simulink model "complementary_controller"  (R2013a)
settings: Solver=ode3  StartTime=0.0  StopTime=15  FixedStep=0.004  RelTol=1e-3
undefined symbols (not defined in the file or in its folder): DiscIntNeverNeededParam, sigbuilder_block
libraries: simulink x3
settings Model: Creator=Matthias  LastModifiedBy=Matthias
settings OptimizationCC: InlineParams=on  InlineInvariantSignals=on  EnhancedBackFolding=on  EfficientFloat2IntCast=on
settings HardwareCC: ProdLargestAtomicInteger=Long  ProdLargestAtomicFloat=Double  ProdHWDeviceType=ARM Compatible->ARM Cortex
settings ModelReferenceCC: UpdateModelReferenceTargets=IfOutOfDate
settings SFSimCC: SFSimEcho=off
settings RTWCC: GenCodeOnly=on  GenerateMakefile=off  RTWCompilerOptimization=On  CheckMdlBeforeBuild=Warning
settings GRTTargetCC: MatFileLogging=off  SupportNonFinite=off

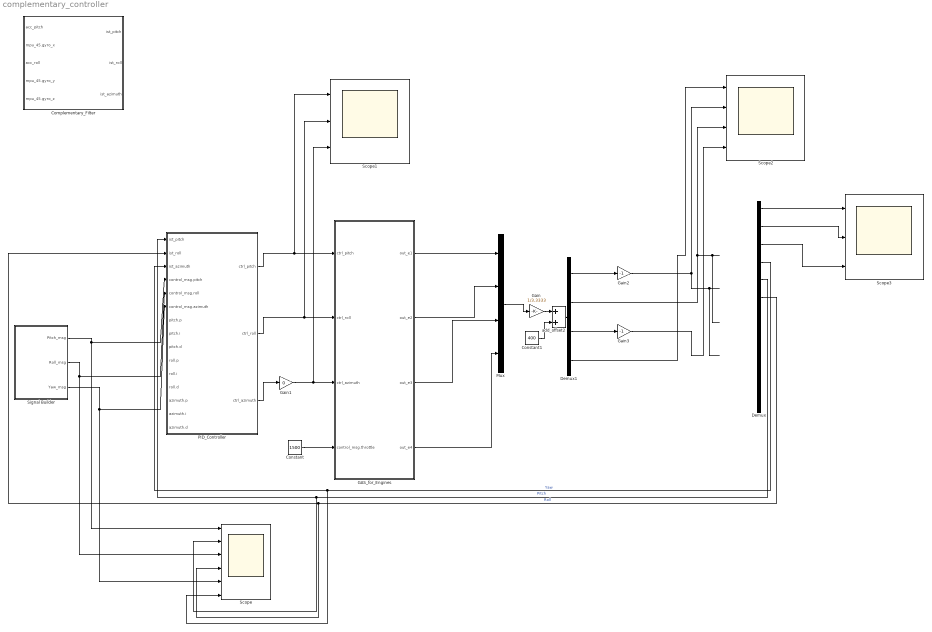
== system complementary_controller ==
  Complementary_Filter : Subsystem
  Constant : Constant  Value=1500
  Constant1 : Constant  Value=400
  Demux : Demux  Outputs=12
  Demux1 : Demux
  GAS_for_Engines : Subsystem
  Gain : Gain  Gain=1/3.3333
  Gain1 : Gain  Gain=0
  Gain2 : Gain  Gain=-1
  Gain3 : Gain  Gain=-1
  Mux : Mux
  PID_Controller : Subsystem
  Scope : Scope  NumInputPorts=6
      settings: YMin=0~-0.1~-1~-2.5e-17~-1~-25  YMax=0.8~0.1~1~0~1~0
  Scope1 : Scope  NumInputPorts=3
      settings: YMin=-5~-5~-5  YMax=5~5~5
  Scope2 : Scope  NumInputPorts=4
      settings: YMin=850.004~-850.005~850.004~-850.005  YMax=850.005~-850.004~850.005~-850.004  SaveName=ScopeData2
  Scope3 : Scope  NumInputPorts=3
      settings: YMin=-18~-7~-0.15  YMax=0~0.5~0  SaveName=ScopeData3
  Signal Builder : Subsystem  Tag=STV Subsys  LoadFcn=sigbuilder_block('load');  StartFcn=sigbuilder_block('start');  StopFcn=sigbuilder_block('stop');  ClipboardFcn=sigbuilder_block('clipboard');  mask(Sigbuilder block){}
      mask help: Simulink:masks:SigbuilderBlock_MD
      mask init:
      | if ~strcmp(get_param(bdroot(gcbh),'SimulationStatus'),'stopped') tuvar = sigbuilder_block('maskInit'); end
      settings: CopyFcn=sigbuilder_block('copy');  DeleteFcn=sigbuilder_block('delete');  ModelCloseFcn=sigbuilder_block('modelClose');  PreSaveFcn=sigbuilder_block('preSave');  PauseFcn=sigbuilder_block('pause');  ContinueFcn=sigbuilder_block('continue');  NameChangeFcn=sigbuilder_block('namechange');  OpenFcn=sigbuilder_block('open',[44.25 171 550.5 399.75 ]);  CloseFcn=sigbuilder_block('close');
      mask Display: plot(0, 0, 100, 100,[2, 2, 32, 32, 2], [68, 8, 8, 68, 68],[32, 2], [38, 38], [32, 19, 2],[53, 60, 44], [32, 17, 17, 2],[16, 16, 31, 31]);txt = getActiveGroup(gcbh);text(2, 100, txt,'verticalAlignment', 'top');
  add_offset2 : Sum
  wires:
  PID_Controller/1(ctrl_pitch) -> Scope1/1, GAS_for_Engines/1(ctrl_pitch)
  PID_Controller/2(ctrl_roll) -> Scope1/2, GAS_for_Engines/2(ctrl_roll)
  PID_Controller/3(ctrl_azimuth) -> Gain1/1
  ? -> Demux/1
  Demux/4 -> Scope/6, PID_Controller/3(ist_azimuth)  "Yaw"
  Demux/5 -> Scope/2, PID_Controller/1(ist_pitch)  "Pitch"
  Demux/6 -> PID_Controller/2(ist_roll), Scope/4  "Roll"
  Signal Builder/1(Pitch_msg) -> Scope/1, PID_Controller/4(control_msg.pitch)
  Signal Builder/2(Roll_msg) -> Scope/3, PID_Controller/5(control_msg.roll)
  Signal Builder/3(Yaw_msg) -> Scope/5, PID_Controller/6(control_msg.azimuth)
  Constant/1 -> GAS_for_Engines/4(control_msg.throttle)
  Gain/1 -> add_offset2/1
  add_offset2/1 -> Demux1/1
  Constant1/1 -> add_offset2/2
  GAS_for_Engines/2(out_e2) -> Mux/2
  Mux/1 -> Gain/1
  GAS_for_Engines/3(out_e3) -> Mux/3
  GAS_for_Engines/4(out_e4) -> Mux/4
  Demux1/1 -> Gain2/1
  Demux1/2 -> Scope2/3
  Demux1/3 -> Gain3/1
  Demux1/4 -> Scope2/1
  Demux/1 -> Scope3/1
  Demux/2 -> Scope3/2
  Demux/3 -> Scope3/3
  Gain1/1 -> Scope1/3, GAS_for_Engines/3(ctrl_azimuth)
  GAS_for_Engines/1(out_e1) -> Mux/1
  Gain3/1 -> Scope2/4
  Gain2/1 -> Scope2/2

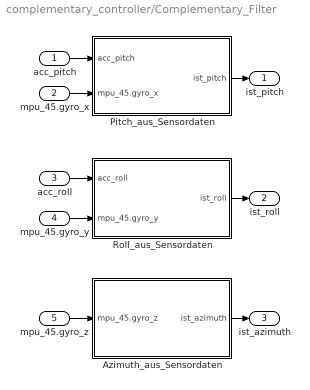
== system complementary_controller/Complementary_Filter ==
  acc_pitch : Inport
  mpu_45.gyro_x : Inport  Port=2
  acc_roll : Inport  Port=3
  mpu_45.gyro_y : Inport  Port=4
  mpu_45.gyro_z : Inport  Port=5
  Azimuth_aus_Sensordaten : Subsystem
  Pitch_aus_Sensordaten : Subsystem
  Roll_aus_Sensordaten : Subsystem
  ist_pitch : Outport
  ist_roll : Outport  Port=2
  ist_azimuth : Outport  Port=3
  wires:
  acc_pitch/1 -> Pitch_aus_Sensordaten/1(acc_pitch)
  mpu_45.gyro_x/1 -> Pitch_aus_Sensordaten/2(mpu_45.gyro_x)
  Roll_aus_Sensordaten/1(ist_roll) -> ist_roll/1
  Azimuth_aus_Sensordaten/1(ist_azimuth) -> ist_azimuth/1
  Pitch_aus_Sensordaten/1(ist_pitch) -> ist_pitch/1
  mpu_45.gyro_y/1 -> Roll_aus_Sensordaten/2(mpu_45.gyro_y)
  acc_roll/1 -> Roll_aus_Sensordaten/1(acc_roll)
  mpu_45.gyro_z/1 -> Azimuth_aus_Sensordaten/1(mpu_45.gyro_z)

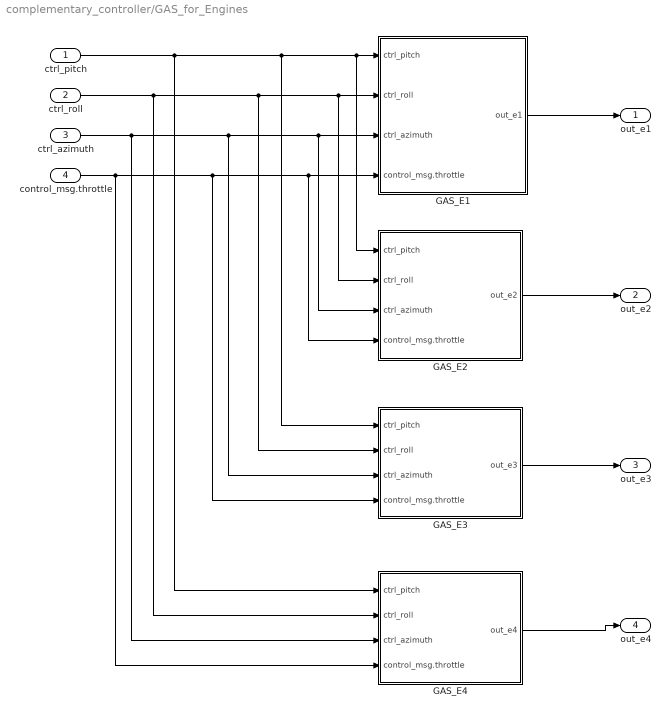
== system complementary_controller/GAS_for_Engines ==
  ctrl_pitch : Inport
  ctrl_roll : Inport  Port=2
  ctrl_azimuth : Inport  Port=3
  control_msg.throttle : Inport  Port=4
  GAS_E1 : Subsystem
  GAS_E2 : Subsystem
  GAS_E3 : Subsystem
  GAS_E4 : Subsystem
  out_e1 : Outport
  out_e2 : Outport  Port=2
  out_e3 : Outport  Port=3
  out_e4 : Outport  Port=4
  wires:
  ctrl_pitch/1 -> GAS_E4/1(ctrl_pitch), GAS_E3/1(ctrl_pitch), GAS_E2/1(ctrl_pitch), GAS_E1/1(ctrl_pitch)
  GAS_E1/1(out_e1) -> out_e1/1
  GAS_E2/1(out_e2) -> out_e2/1
  ctrl_roll/1 -> GAS_E4/2(ctrl_roll), GAS_E2/2(ctrl_roll), GAS_E1/2(ctrl_roll), GAS_E3/2(ctrl_roll)
  GAS_E3/1(out_e3) -> out_e3/1
  ctrl_azimuth/1 -> GAS_E2/3(ctrl_azimuth), GAS_E1/3(ctrl_azimuth), GAS_E3/3(ctrl_azimuth), GAS_E4/3(ctrl_azimuth)
  GAS_E4/1(out_e4) -> out_e4/1
  control_msg.throttle/1 -> GAS_E4/4(control_msg.throttle), GAS_E3/4(control_msg.throttle), GAS_E1/4(control_msg.throttle), GAS_E2/4(control_msg.throttle)

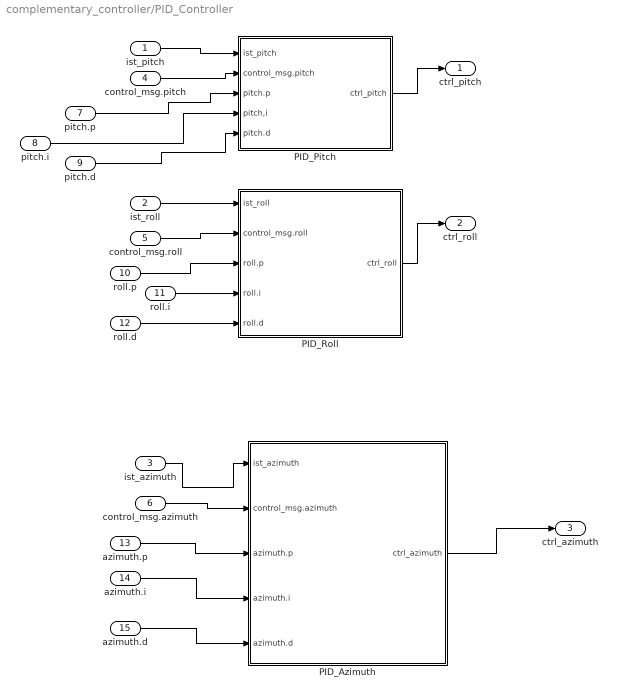
== system complementary_controller/PID_Controller ==
  ist_pitch : Inport
  ist_roll : Inport  Port=2
  ist_azimuth : Inport  Port=3
  control_msg.pitch : Inport  Port=4
  control_msg.roll : Inport  Port=5
  control_msg.azimuth : Inport  Port=6
  pitch.p : Inport  Port=7
  pitch.i : Inport  Port=8
  pitch.d : Inport  Port=9
  roll.p : Inport  Port=10
  roll.i : Inport  Port=11
  roll.d : Inport  Port=12
  azimuth.p : Inport  Port=13
  azimuth.i : Inport  Port=14
  azimuth.d : Inport  Port=15
  PID_Azimuth : Subsystem
  PID_Pitch : Subsystem
  PID_Roll : Subsystem
  ctrl_pitch : Outport
  ctrl_roll : Outport  Port=2
  ctrl_azimuth : Outport  Port=3
  wires:
  ist_pitch/1 -> PID_Pitch/1(ist_pitch)
  PID_Pitch/1(ctrl_pitch) -> ctrl_pitch/1
  control_msg.pitch/1 -> PID_Pitch/2(control_msg.pitch)
  ist_azimuth/1 -> PID_Azimuth/1(ist_azimuth)
  control_msg.azimuth/1 -> PID_Azimuth/2(control_msg.azimuth)
  PID_Azimuth/1(ctrl_azimuth) -> ctrl_azimuth/1
  PID_Roll/1(ctrl_roll) -> ctrl_roll/1
  ist_roll/1 -> PID_Roll/1(ist_roll)
  control_msg.roll/1 -> PID_Roll/2(control_msg.roll)
  pitch.p/1 -> PID_Pitch/3(pitch.p)
  pitch.i/1 -> PID_Pitch/4(pitch,i)
  pitch.d/1 -> PID_Pitch/5(pitch.d)
  roll.p/1 -> PID_Roll/3(roll.p)
  roll.d/1 -> PID_Roll/5(roll.d)
  roll.i/1 -> PID_Roll/4(roll.i)
  azimuth.p/1 -> PID_Azimuth/3(azimuth.p)
  azimuth.i/1 -> PID_Azimuth/4(azimuth.i)
  azimuth.d/1 -> PID_Azimuth/5(azimuth.d)

== system complementary_controller/Signal Builder ==
  Demux : Demux  Tag=STV Demux  Outputs=3
  FromWs : FromWorkspace  Tag=STV FromWs  VariableName=tuvar  SampleTime=0
      SigBuilderData=|
      | common.afterFinalStr = 'Extrapolate'
      | common.sampleTime = 0
      | dataSet.timeRange = [0 10]
      | dataSet.name = 'Group 1'
      | sbobj.Groups.Name = 'Group 1'
      | sbobj.Groups.Signals(1).Name = 'Pitch_msg'
      | sbobj.Groups.Signals(1).XData = [0 3 3 6 6 10]
      | sbobj.Groups.Signals(1).YData = [0 0 0.99 0.99 0 0]
      | sbobj.Groups.Signals(2).Name = 'Roll_msg'
      | sbobj.Groups.Signals(2).XData = [0 1.28 6.68 10]
      | sbobj.Groups.Signals(2).YData = [0 0 0 0]
      | sbobj.Groups.Signals(3).Name = 'Yaw_msg'
      | sbobj.Groups.Signals(3).XData = [0 1.56 2.72 10]
      | sbobj.Groups.Signals(3).YData = [0 0 0 0]
  Pitch_msg : Outport  Tag=STV Outport
  Roll_msg : Outport  Tag=STV Outport  Port=2
  Yaw_msg : Outport  Tag=STV Outport  Port=3
  wires:
  Demux/1 -> Pitch_msg/1
  FromWs/1 -> Demux/1
  Demux/2 -> Roll_msg/1
  Demux/3 -> Yaw_msg/1

== system complementary_controller/Complementary_Filter/Azimuth_aus_Sensordaten ==
  mpu_45.gyro_z : Inport
  Discrete-Time Integrator : DiscreteIntegrator  InitialConditionMode=State only (most efficient)  SampleTime=0.004  SaturateOnIntegerOverflow=on  LimitOutput=on  UpperSaturationLimit=0.5*10^18  LowerSaturationLimit=-0.5*10^18  ICPrevOutput=DiscIntNeverNeededParam  ICPrevScaledInput=DiscIntNeverNeededParam
  ist_azimuth : Outport
  wires:
  mpu_45.gyro_z/1 -> Discrete-Time Integrator/1
  Discrete-Time Integrator/1 -> ist_azimuth/1

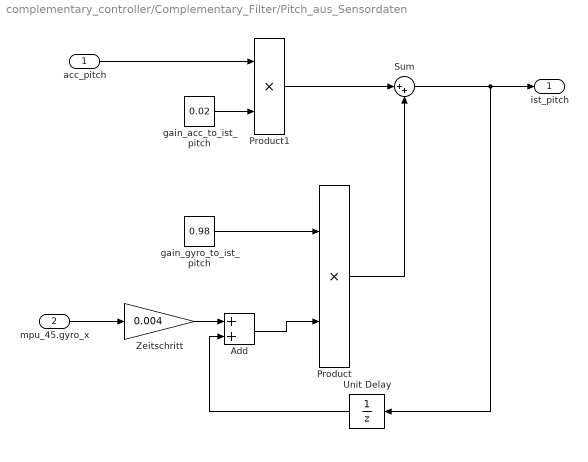
== system complementary_controller/Complementary_Filter/Pitch_aus_Sensordaten ==
  acc_pitch : Inport
  mpu_45.gyro_x : Inport  Port=2
  Add : Sum
  Product : Product
  Product1 : Product
  Sum : Sum  Inputs=|++
  Unit Delay : UnitDelay  SampleTime=-1
  Zeitschritt : Gain  Gain=0.004
  gain_acc_to_ist_pitch : Constant  Value=0.02
  gain_gyro_to_ist_pitch : Constant  Value=0.98
  ist_pitch : Outport
  wires:
  mpu_45.gyro_x/1 -> Zeitschritt/1
  gain_acc_to_ist_pitch/1 -> Product1/2
  acc_pitch/1 -> Product1/1
  Product1/1 -> Sum/1
  gain_gyro_to_ist_pitch/1 -> Product/1
  Sum/1 -> Unit Delay/1, ist_pitch/1
  Unit Delay/1 -> Add/2
  Zeitschritt/1 -> Add/1
  Add/1 -> Product/2
  Product/1 -> Sum/2

== system complementary_controller/Complementary_Filter/Roll_aus_Sensordaten ==
  acc_roll : Inport
  mpu_45.gyro_y : Inport  Port=2
  Product2 : Product
  Product3 : Product
  Sum1 : Sum  Inputs=|++
  Sum2 : Sum  Inputs=|++
  Unit Delay : UnitDelay  SampleTime=-1
  Zeitschritt : Gain  Gain=0.004
  gain_acc_to_ist_roll : Constant  Value=0.02
  gain_gyro_to_ist_roll : Constant  Value=0.98
  ist_roll : Outport
  wires:
  Zeitschritt/1 -> Sum2/1
  gain_acc_to_ist_roll/1 -> Product3/2
  Product3/1 -> Sum1/1
  Product2/1 -> Sum1/2
  Sum2/1 -> Product2/2
  gain_gyro_to_ist_roll/1 -> Product2/1
  Sum1/1 -> ist_roll/1, Unit Delay/1
  Unit Delay/1 -> Sum2/2
  acc_roll/1 -> Product3/1
  mpu_45.gyro_y/1 -> Zeitschritt/1

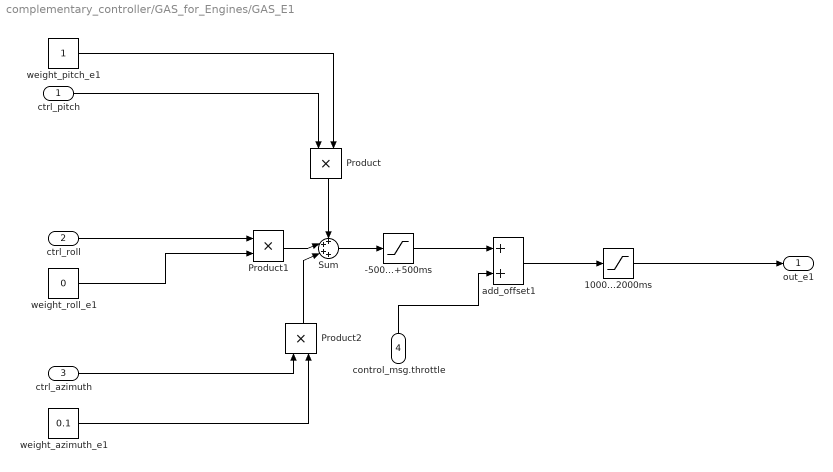
== system complementary_controller/GAS_for_Engines/GAS_E1 ==
  ctrl_pitch : Inport
  ctrl_roll : Inport  Port=2
  ctrl_azimuth : Inport  Port=3
  control_msg.throttle : Inport  Port=4
  -500...+500ms : Saturate  UpperLimit=500  LowerLimit=-500
  1000...2000ms : Saturate  UpperLimit=2000  LowerLimit=1000
  Product : Product
  Product1 : Product
  Product2 : Product
  Sum : Sum  Inputs=++++
  add_offset1 : Sum
  weight_azimuth_e1 : Constant  Value=0.1
  weight_pitch_e1 : Constant
  weight_roll_e1 : Constant  Value=0
  out_e1 : Outport
  wires:
  Product/1 -> Sum/1
  Product1/1 -> Sum/2
  Product2/1 -> Sum/3
  ctrl_roll/1 -> Product1/1
  ctrl_pitch/1 -> Product/1
  ctrl_azimuth/1 -> Product2/1
  weight_roll_e1/1 -> Product1/2
  weight_pitch_e1/1 -> Product/2
  weight_azimuth_e1/1 -> Product2/2
  Sum/1 -> -500...+500ms/1
  control_msg.throttle/1 -> add_offset1/2
  -500...+500ms/1 -> add_offset1/1
  add_offset1/1 -> 1000...2000ms/1
  1000...2000ms/1 -> out_e1/1

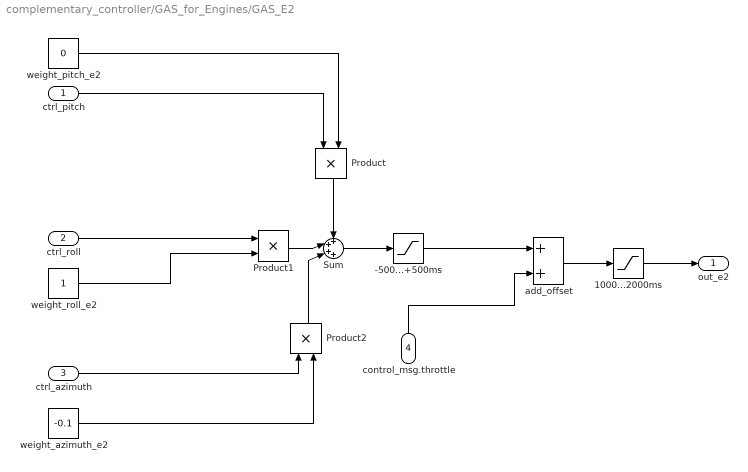
== system complementary_controller/GAS_for_Engines/GAS_E2 ==
  ctrl_pitch : Inport
  ctrl_roll : Inport  Port=2
  ctrl_azimuth : Inport  Port=3
  control_msg.throttle : Inport  Port=4
  -500...+500ms : Saturate  UpperLimit=500  LowerLimit=-500
  1000...2000ms : Saturate  UpperLimit=2000  LowerLimit=1000
  Product : Product
  Product1 : Product
  Product2 : Product
  Sum : Sum  Inputs=++++
  add_offset : Sum
  weight_azimuth_e2 : Constant  Value=-0.1
  weight_pitch_e2 : Constant  Value=0
  weight_roll_e2 : Constant
  out_e2 : Outport
  wires:
  Product/1 -> Sum/1
  Product1/1 -> Sum/2
  Product2/1 -> Sum/3
  ctrl_roll/1 -> Product1/1
  ctrl_pitch/1 -> Product/1
  ctrl_azimuth/1 -> Product2/1
  weight_roll_e2/1 -> Product1/2
  weight_pitch_e2/1 -> Product/2
  weight_azimuth_e2/1 -> Product2/2
  Sum/1 -> -500...+500ms/1
  control_msg.throttle/1 -> add_offset/2
  -500...+500ms/1 -> add_offset/1
  add_offset/1 -> 1000...2000ms/1
  1000...2000ms/1 -> out_e2/1

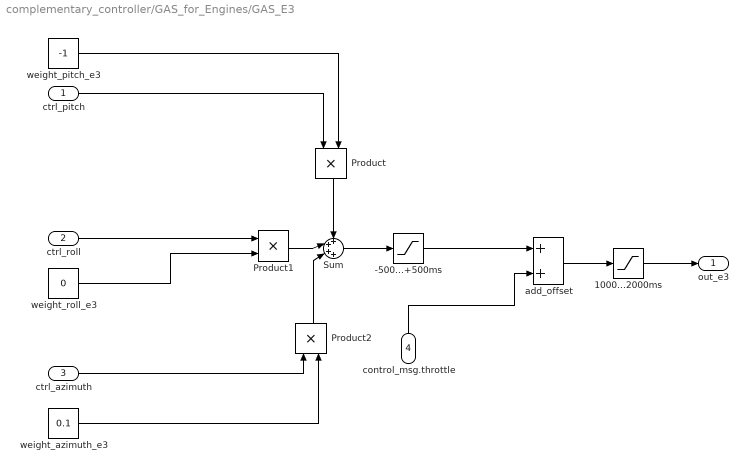
== system complementary_controller/GAS_for_Engines/GAS_E3 ==
  ctrl_pitch : Inport
  ctrl_roll : Inport  Port=2
  ctrl_azimuth : Inport  Port=3
  control_msg.throttle : Inport  Port=4
  -500...+500ms : Saturate  UpperLimit=500  LowerLimit=-500
  1000...2000ms : Saturate  UpperLimit=2000  LowerLimit=1000
  Product : Product
  Product1 : Product
  Product2 : Product
  Sum : Sum  Inputs=++++
  add_offset : Sum
  weight_azimuth_e3 : Constant  Value=0.1
  weight_pitch_e3 : Constant  Value=-1
  weight_roll_e3 : Constant  Value=0
  out_e3 : Outport
  wires:
  Product/1 -> Sum/1
  Sum/1 -> -500...+500ms/1
  Product1/1 -> Sum/2
  Product2/1 -> Sum/3
  ctrl_roll/1 -> Product1/1
  ctrl_pitch/1 -> Product/1
  ctrl_azimuth/1 -> Product2/1
  weight_roll_e3/1 -> Product1/2
  weight_pitch_e3/1 -> Product/2
  weight_azimuth_e3/1 -> Product2/2
  control_msg.throttle/1 -> add_offset/2
  -500...+500ms/1 -> add_offset/1
  add_offset/1 -> 1000...2000ms/1
  1000...2000ms/1 -> out_e3/1

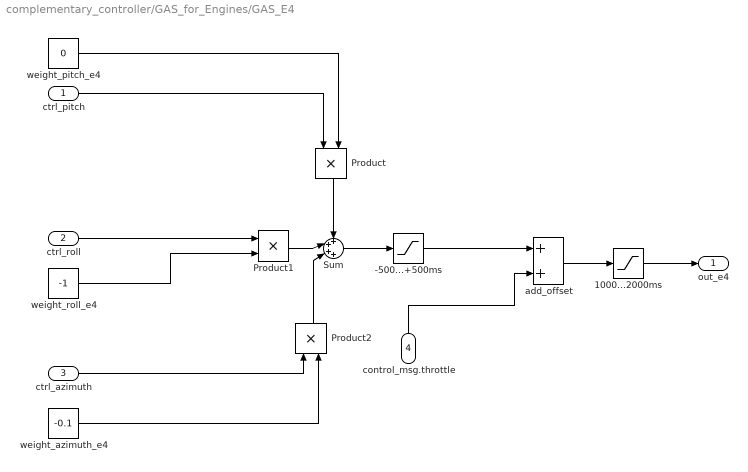
== system complementary_controller/GAS_for_Engines/GAS_E4 ==
  ctrl_pitch : Inport
  ctrl_roll : Inport  Port=2
  ctrl_azimuth : Inport  Port=3
  control_msg.throttle : Inport  Port=4
  -500...+500ms : Saturate  UpperLimit=500  LowerLimit=-500
  1000...2000ms : Saturate  UpperLimit=2000  LowerLimit=1000
  Product : Product
  Product1 : Product
  Product2 : Product
  Sum : Sum  Inputs=++++
  add_offset : Sum
  weight_azimuth_e4 : Constant  Value=-0.1
  weight_pitch_e4 : Constant  Value=0
  weight_roll_e4 : Constant  Value=-1
  out_e4 : Outport
  wires:
  Product/1 -> Sum/1
  Product1/1 -> Sum/2
  Product2/1 -> Sum/3
  ctrl_roll/1 -> Product1/1
  ctrl_pitch/1 -> Product/1
  ctrl_azimuth/1 -> Product2/1
  weight_roll_e4/1 -> Product1/2
  weight_pitch_e4/1 -> Product/2
  weight_azimuth_e4/1 -> Product2/2
  Sum/1 -> -500...+500ms/1
  control_msg.throttle/1 -> add_offset/2
  -500...+500ms/1 -> add_offset/1
  add_offset/1 -> 1000...2000ms/1
  1000...2000ms/1 -> out_e4/1

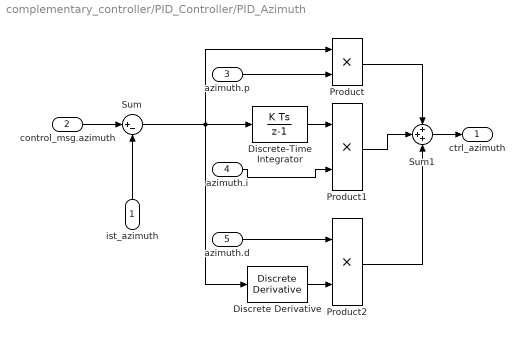
== system complementary_controller/PID_Controller/PID_Azimuth ==
  ist_azimuth : Inport
  control_msg.azimuth : Inport  Port=2
  azimuth.p : Inport  Port=3
  azimuth.i : Inport  Port=4
  azimuth.d : Inport  Port=5
  Discrete Derivative : simulink/Discrete/Discrete Derivative  gainval=1.0  ICPrevScaledInput=0.0  InputProcessing=Inherited  OutMin=[]  OutMax=[]  OutDataType=fixdt(1, 16)  OutScaling=2^-10  DoSatur=off
  Discrete-Time Integrator : DiscreteIntegrator  SampleTime=0.004  SaturateOnIntegerOverflow=on  LimitOutput=on  UpperSaturationLimit=0.5*10^18  LowerSaturationLimit=-0.5*10^18  ICPrevOutput=DiscIntNeverNeededParam  ICPrevScaledInput=DiscIntNeverNeededParam
  Product : Product
  Product1 : Product
  Product2 : Product
  Sum : Sum  Inputs=|+-
  Sum1 : Sum  Inputs=+++
  ctrl_azimuth : Outport
  wires:
  ist_azimuth/1 -> Sum/2
  control_msg.azimuth/1 -> Sum/1
  Sum1/1 -> ctrl_azimuth/1
  Sum/1 -> Discrete Derivative/1, Discrete-Time Integrator/1, Product/1
  azimuth.p/1 -> Product/2
  Product/1 -> Sum1/1
  Product1/1 -> Sum1/2
  Discrete-Time Integrator/1 -> Product1/1
  azimuth.i/1 -> Product1/2
  Product2/1 -> Sum1/3
  Discrete Derivative/1 -> Product2/2
  azimuth.d/1 -> Product2/1

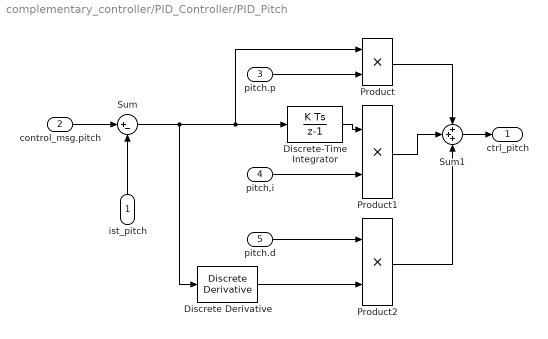
== system complementary_controller/PID_Controller/PID_Pitch ==
  ist_pitch : Inport
  control_msg.pitch : Inport  Port=2
  pitch.p : Inport  Port=3
  pitch,i : Inport  Port=4
  pitch.d : Inport  Port=5
  Discrete Derivative : simulink/Discrete/Discrete Derivative  gainval=1.0  ICPrevScaledInput=0.0  InputProcessing=Inherited  OutMin=[]  OutMax=[]  OutDataType=fixdt(1, 16)  OutScaling=2^-10  DoSatur=off
  Discrete-Time Integrator : DiscreteIntegrator  SampleTime=0.004  SaturateOnIntegerOverflow=on  LimitOutput=on  UpperSaturationLimit=0.5*10^18  LowerSaturationLimit=-0.5*10^18  ICPrevOutput=DiscIntNeverNeededParam  ICPrevScaledInput=DiscIntNeverNeededParam
  Product : Product
  Product1 : Product
  Product2 : Product
  Sum : Sum  Inputs=|+-
  Sum1 : Sum  Inputs=+++
  ctrl_pitch : Outport
  wires:
  ist_pitch/1 -> Sum/2
  control_msg.pitch/1 -> Sum/1
  Sum1/1 -> ctrl_pitch/1
  Sum/1 -> Discrete Derivative/1, Product/1, Discrete-Time Integrator/1
  pitch.p/1 -> Product/2
  Product/1 -> Sum1/1
  Product1/1 -> Sum1/2
  Discrete-Time Integrator/1 -> Product1/1
  pitch,i/1 -> Product1/2
  Product2/1 -> Sum1/3
  pitch.d/1 -> Product2/1
  Discrete Derivative/1 -> Product2/2

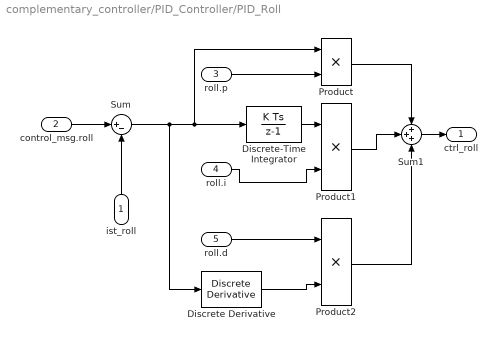
== system complementary_controller/PID_Controller/PID_Roll ==
  ist_roll : Inport
  control_msg.roll : Inport  Port=2
  roll.p : Inport  Port=3
  roll.i : Inport  Port=4
  roll.d : Inport  Port=5
  Discrete Derivative : simulink/Discrete/Discrete Derivative  gainval=1.0  ICPrevScaledInput=0.0  InputProcessing=Inherited  OutMin=[]  OutMax=[]  OutDataType=fixdt(1, 16)  OutScaling=2^-10  DoSatur=off
  Discrete-Time Integrator : DiscreteIntegrator  SampleTime=0.004  SaturateOnIntegerOverflow=on  LimitOutput=on  UpperSaturationLimit=0.5*10^18  LowerSaturationLimit=-0.5*10^18  ICPrevOutput=DiscIntNeverNeededParam  ICPrevScaledInput=DiscIntNeverNeededParam
  Product : Product
  Product1 : Product
  Product2 : Product
  Sum : Sum  Inputs=|+-
  Sum1 : Sum  Inputs=+++
  ctrl_roll : Outport
  wires:
  ist_roll/1 -> Sum/2
  control_msg.roll/1 -> Sum/1
  Sum1/1 -> ctrl_roll/1
  Sum/1 -> Discrete Derivative/1, Discrete-Time Integrator/1, Product/1
  roll.p/1 -> Product/2
  Product/1 -> Sum1/1
  Product1/1 -> Sum1/2
  Discrete-Time Integrator/1 -> Product1/1
  roll.i/1 -> Product1/2
  Product2/1 -> Sum1/3
  roll.d/1 -> Product2/1
  Discrete Derivative/1 -> Product2/2
